simulink model "Bahnschwingung"  (R2021b)
settings: Solver=ode4  StartTime=0.0  StopTime=1000  FixedStep=0.002  RelTol=1e-3
undefined symbols (not defined in the file): BFZ, ENV
settings Model: Creator=jonih  LastModifiedBy=jonih

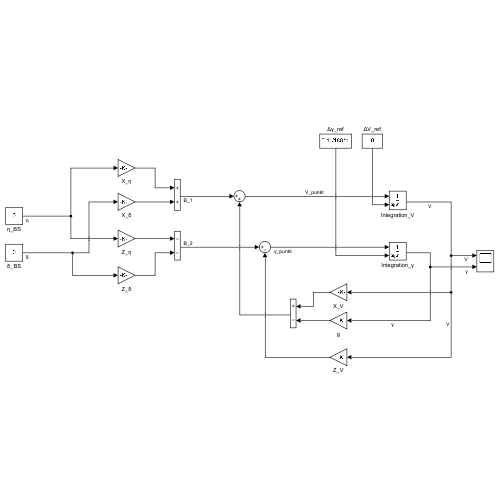
[thumbnail: Simulink's stored preview of the top-level diagram]
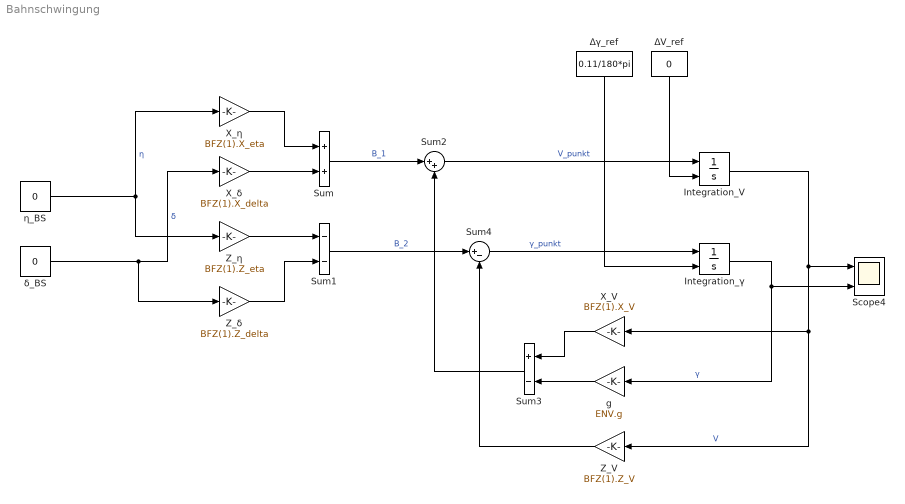
== system Bahnschwingung ==
  Integration_V : Integrator  InitialConditionSource=external
  Integration_γ : Integrator  InitialConditionSource=external
  Scope4 : Scope  NumInputPorts=2
  Sum : Sum
  Sum1 : Sum  Inputs=--
  Sum2 : Sum  Inputs=|++
  Sum3 : Sum  Inputs=+-
  Sum4 : Sum  Inputs=|+-
  X_V : Gain  Gain=BFZ(1).X_V
  X_δ : Gain  Gain=BFZ(1).X_delta
  X_η : Gain  Gain=BFZ(1).X_eta
  Z_V : Gain  Gain=BFZ(1).Z_V
  Z_δ : Gain  Gain=BFZ(1).Z_delta
  Z_η : Gain  Gain=BFZ(1).Z_eta
  g : Gain  Gain=ENV.g
  ΔV_ref : Constant  Value=0
  Δγ_ref : Constant  Value=0.11/180*pi
  δ_BS : Constant  Value=0
  η_BS : Constant  Value=0
  wires:
  Sum2/1 -> Integration_V/1  "V_punkt"
  Sum/1 -> Sum2/1  "B_1"
  ΔV_ref/1 -> Integration_V/2
  η_BS/1 -> Z_η/1, X_η/1  "η"
  Z_V/1 -> Sum4/2
  Integration_V/1 -> Scope4/1, Z_V/1, X_V/1  "V"
  Integration_γ/1 -> g/1, Scope4/2  "γ"
  δ_BS/1 -> X_δ/1, Z_δ/1  "δ"
  Sum1/1 -> Sum4/1  "B_2"
  Z_δ/1 -> Sum1/2
  X_δ/1 -> Sum/2
  Z_η/1 -> Sum1/1
  X_η/1 -> Sum/1
  X_V/1 -> Sum3/1
  g/1 -> Sum3/2
  Δγ_ref/1 -> Integration_γ/2
  Sum3/1 -> Sum2/2
  Sum4/1 -> Integration_γ/1  "γ_punkt"
